simulink model "pll03"  (Simulink 8.1)
settings: Solver=ode45  StartTime=0.0  StopTime=10  MaxStep=0.0001  RelTol=1e-3
undefined symbols (not defined in the file or in its folder): fdesignblkfcn, gcbh
libraries: commsynccomp2 x1, commnoisgen2 x1, simulink x1
settings Model: Creator=my88899  LastModifiedBy=my88899
settings DataIOCC: SignalLoggingSaveFormat=Dataset
settings OptimizationCC: ExpressionDepthLimit=128
settings DebuggingCC: FcnCallInpInsideContextMsg=EnableAllAsError
settings GRTTargetCC: CombineOutputUpdateFcns=on  GRTInterface=off

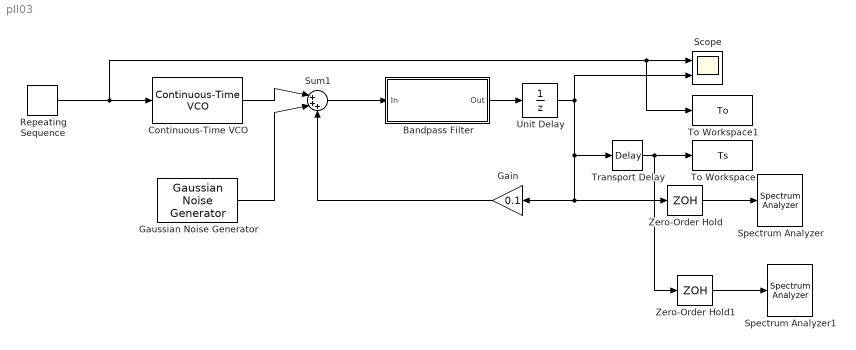
== system pll03 ==
  Bandpass Filter : Subsystem  DialogController=fdesignblkfcn  DialogControllerArgs=DataTag1  InitFcn=fdesignblkfcn(gcbh, {'InitFcn'});  mask(Bandpass Filter){}
      mask help: Design a bandpass filter
      settings: CopyFcn=fdesignblkfcn(gcbh, {'CopyFcn'});
      mask Help: helpview(mapfilelocation('dsp'), 'dspbandpassfilter');
      mask Display: disp('Bandpass');
  Continuous-Time VCO : commsynccomp2/Continuous-Time VCO  Ac=5  Fc=100  Kc=100  Ph=0
  Gain : Gain  Gain=0.1
  Gaussian Noise Generator : commnoisgen2/Gaussian Noise Generator  m=0  d=1  s=2333  Ts=0.1  frameBased=off  sampPerFrame=1  orient=off  outDataType=double
  Repeating Sequence : simulink/Sources/Repeating Sequence  rep_seq_t=[0 1]  rep_seq_y=[0 5]
  Scope : Scope  NumInputPorts=2
      settings: TimeRange=0.1038961038961048  YMin=5.645~-5  YMax=5.7~5  MaxDataPoints=100000
  Spectrum Analyzer : SpectrumAnalyzer
      settings: CopyFcn=scopeextensions.ScopeBlock.callback(gcbh, 'onBlockCopy', gcbh);  DeleteFcn=scopeextensions.ScopeBlock.callback(gcbh, 'onBlockDelete');  PreSaveFcn=scopeextensions.ScopeBlock.callback(gcbh, 'onModelSave');  NameChangeFcn=scopeextensions.ScopeBlock.callback(gcbh, 'onBlockRename');  CloseFcn=scopeextensions.ScopeBlock.callback(gcbh, 'onBlockClose');  PreDeleteFcn=scopeextensions.ScopeBlock.callback(gcbh, 'onBlockPreDelete');
  Spectrum Analyzer1 : SpectrumAnalyzer
      settings: CopyFcn=scopeextensions.ScopeBlock.callback(gcbh, 'onBlockCopy', gcbh);  DeleteFcn=scopeextensions.ScopeBlock.callback(gcbh, 'onBlockDelete');  PreSaveFcn=scopeextensions.ScopeBlock.callback(gcbh, 'onModelSave');  NameChangeFcn=scopeextensions.ScopeBlock.callback(gcbh, 'onBlockRename');  CloseFcn=scopeextensions.ScopeBlock.callback(gcbh, 'onBlockClose');  PreDeleteFcn=scopeextensions.ScopeBlock.callback(gcbh, 'onBlockPreDelete');
  Sum1 : Sum  Inputs=|+++
  To Workspace : ToWorkspace  VariableName=Ts  SampleTime=-1  SaveFormat=Timeseries
  To Workspace1 : ToWorkspace  VariableName=To  SampleTime=-1  SaveFormat=Timeseries
  Transport Delay : TransportDelay  DelayTime=0.5
  Unit Delay : UnitDelay  SampleTime=-1
  Zero-Order Hold : ZeroOrderHold  SampleTime=0.01
  Zero-Order Hold1 : ZeroOrderHold  SampleTime=0.01
  wires:
  Repeating Sequence/1 -> To Workspace1/1, Scope/1, Continuous-Time VCO/1
  Zero-Order Hold/1 -> Spectrum Analyzer/1
  Gain/1 -> Sum1/3
  Bandpass Filter/1(Out) -> Unit Delay/1
  Sum1/1 -> Bandpass Filter/1(In)
  Continuous-Time VCO/1 -> Sum1/1
  Gaussian Noise Generator/1 -> Sum1/2
  Unit Delay/1 -> Scope/2, Zero-Order Hold/1, Gain/1, Transport Delay/1
  Zero-Order Hold1/1 -> Spectrum Analyzer1/1
  Transport Delay/1 -> To Workspace/1, Zero-Order Hold1/1

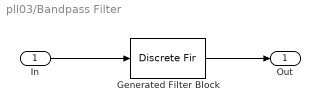
== system pll03/Bandpass Filter ==
  In : Inport
  Generated Filter Block : DiscreteFir  Tag=BlockMethodSubSystem  Coefficients=[-0.0008992291487744296 0.0016414518747943749 0.0031352071842225397 -0.0040707550828814922 -0.0063731852227904111 0.0074874286806090491 0.0098354319566295711 -0.010189316513446216 -0.011302794465874122 0.0096929185841818435 0.0079428653987464216 -0.0031368247881221642 0.0028299878877943137 -0.011508674243001471 -0.022080136219461581 0.034245325424507672 0.048356661648905473 -0.062355369169884239 -0.077503478162593897 0.090687768153125653 0.10353171105844157 -0.11297860084229834 -0.12035866024978455 0.12379360801539134 0.12379360801539134 -0.12035866024978455 -0.11297860084229834 0.10353171105844157 0.090687768153125653 -0.077503478162593897 -0.062355369169884239 0.048356661648905473 0.034245325424507672 -0.022080136219461581 -0.011508674243001471 0.0028299878877943137 -0.0031368247881221642 0.0079428653987464216 0.0096929185841818435 -0.011302794465874122 -0.010189316513446216 0.0098354319566295711 0.0074874286806090491 -0.0063731852227904111 -0.0040707550828814922 0.0031352071842225397 0.0016414518747943749 -0.0008992291487744296]  InputProcessing=Columns as channels (frame based)
  Out : Outport
  wires:
  In/1 -> Generated Filter Block/1
  Generated Filter Block/1 -> Out/1
